simulink model "ARDrone_TrayZ"  (R2020b)
settings: Solver=FixedStepAuto  StartTime=0.0  StopTime=inf  FixedStep=0.001  RelTol=1e-3
PostLoadFcn:
  | load grid_1000m.mat
values from neighbouring files (symbols this model uses):
  D = 1    [Referencias.m]
  dimx = 1000    [grid_1000m.mat]    (also in grid_100m.mat = 100)
  dimy = 1000    [grid_1000m.mat]    (also in grid_100m.mat = 100)
  No = 10    [Referencias.m]
  np = length(Xp)    [Referencias.m]
  T = 0.05    [Referencias.m]
  X = [0 2.5 5 5 5 2.5 0 0]    [Referencias.m]
  Xp = - ( r * cos(th) + x)    [Referencias.m]
  Y = [0 0 0 2.5 5 5 5 2.5]    [Referencias.m]
  Yp = - ( r * sin(th) + y)    [Referencias.m]
  Z = [5 5 5 5 5 5 5 5]    [Referencias.m]
  Zp = 0:0.1:20    [Referencias.m]
libraries: sm_lib x31, nesl_utility x19, dspnetwork x2, simulink_extras x1, simulink x1, vrlib x1
(part 2 of 2)

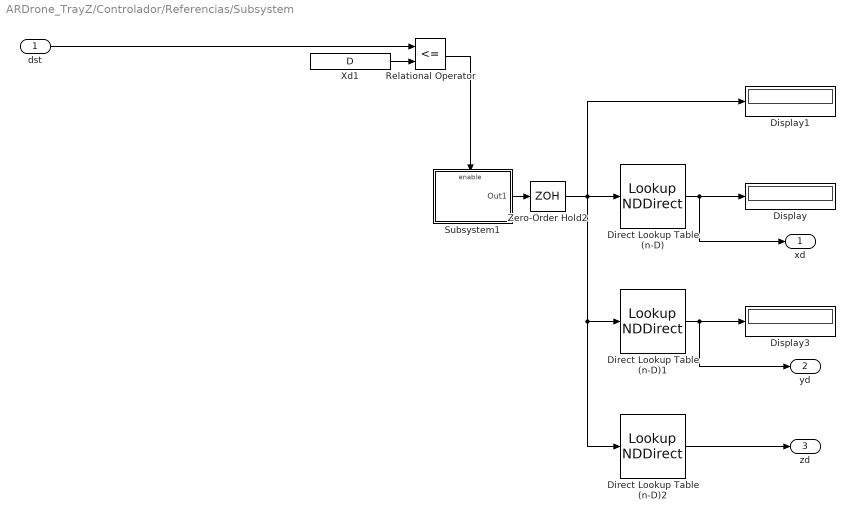
== system ARDrone_TrayZ/Controlador/Referencias/Subsystem ==
  dst : Inport
  Direct Lookup Table (n-D) : LookupNDDirect  NumberOfTableDimensions=1  Table=Xp
  Direct Lookup Table (n-D)1 : LookupNDDirect  NumberOfTableDimensions=1  Table=Yp
  Direct Lookup Table (n-D)2 : LookupNDDirect  NumberOfTableDimensions=1  Table=Zp
  Display : Display
  Display1 : Display
  Display3 : Display
  Relational Operator : RelationalOperator  Operator=<=  OutDataTypeStr=boolean  RndMeth=Nearest
  Subsystem1 : Subsystem
  Xd1 : Constant  Value=D  SampleTime=No*T
  Zero-Order Hold2 : ZeroOrderHold  SampleTime=T
  xd : Outport  VectorParamsAs1DForOutWhenUnconnected=off
  yd : Outport  Port=2  VectorParamsAs1DForOutWhenUnconnected=off
  zd : Outport  Port=3  VectorParamsAs1DForOutWhenUnconnected=off
  wires:
  Relational Operator/1 -> Subsystem1/Enable
  dst/1 -> Relational Operator/1
  Subsystem1/1(Out1) -> Zero-Order Hold2/1
  Direct Lookup Table (n-D)1/1 -> Display3/1, yd/1
  Xd1/1 -> Relational Operator/2
  Direct Lookup Table (n-D)/1 -> Display/1, xd/1
  Zero-Order Hold2/1 -> Direct Lookup Table (n-D)/1, Display1/1, Direct Lookup Table (n-D)2/1, Direct Lookup Table (n-D)1/1
  Direct Lookup Table (n-D)2/1 -> zd/1

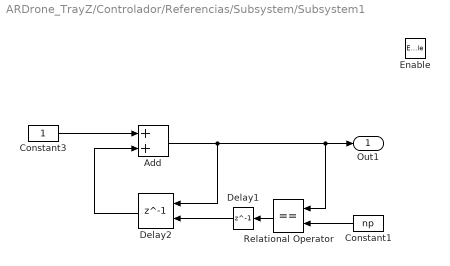
== system ARDrone_TrayZ/Controlador/Referencias/Subsystem/Subsystem1 ==
  Enable : EnablePort
  Add : Sum
  Constant1 : Constant  Value=np  SampleTime=No*T
  Constant3 : Constant  SampleTime=No*T
  Delay1 : Delay  DelayLength=1  InitialCondition=0
  Delay2 : Delay  DelayLength=1  InitialCondition=0  ExternalReset=Rising
      settings: InputPortMap=u0,r5
  Relational Operator : RelationalOperator  Operator===  OutDataTypeStr=boolean  RndMeth=Simplest
  Out1 : Outport  VectorParamsAs1DForOutWhenUnconnected=off
  wires:
  Add/1 -> Relational Operator/1, Out1/1, Delay2/1
  Delay2/1 -> Add/2
  Constant3/1 -> Add/1
  Relational Operator/1 -> Delay1/1
  Constant1/1 -> Relational Operator/2
  Delay1/1 -> Delay2/2
